simulink model "task2"  (R2018a)
settings: Solver=VariableStepAuto  StartTime=0.0  StopTime=0.1  RelTol=1e-3
settings Model: Creator=symih  LastModifiedBy=symih

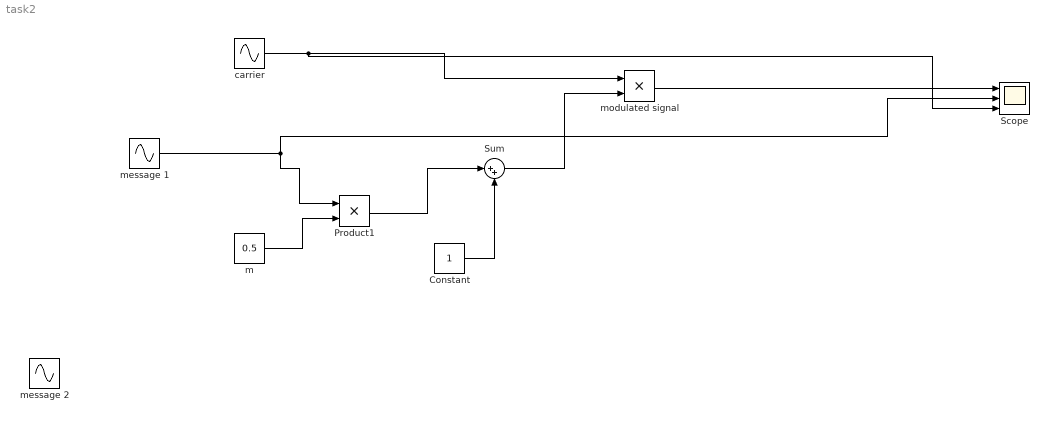
== system task2 ==
  Constant : Constant
  Product1 : Product
  Scope : Scope  NumInputPorts=3
  Sum : Sum  Inputs=|++
  carrier : Sin  Amplitude=21  Frequency=2*pi*6*50*10  Phase=pi/6  SampleTime=0
  m : Constant  Value=0.5
  message 1 : Sin  Amplitude=21  Frequency=2*pi*6*50  Phase=pi/6  SampleTime=0
  message 2 : Sin  Frequency=2*pi*6  Phase=pi/2  SampleTime=0
  modulated signal : Product
  wires:
  Product1/1 -> Sum/1
  Sum/1 -> modulated signal/2
  message 1/1 -> Product1/1, Scope/2
  Constant/1 -> Sum/2
  m/1 -> Product1/2
  carrier/1 -> Scope/3, modulated signal/1
  modulated signal/1 -> Scope/1
